simulink model "LRMate200Experimentor_RobotState"  (R2015b)
settings: Solver=FixedStepDiscrete  StartTime=0.0  StopTime=10.0  FixedStep=si.SolverTimeStep  RelTol=1e-3
model workspace (MATLAB code in the model file):
  | rsi = evalin('base', 'si.ri{1}');
undefined symbols (not defined in the file or in its folder): si
libraries: xpcethercatlib x171
(part 2 of 2)

== system LRMate200Experimentor_RobotState/Not Used/DSA System Variant/DSA System (Robot 2)/EtherCAT DSA CurrentOut ==
  FromDSA J1Current : xpcethercatlib/EtherCAT PDO Receive  Priority=2  sig_name=Box 3 (Degital Servo Adapter).HS-IN-AX01.AX01-HSI03  sig_offset=4968  sig_type=int16  type_size=16  sig_dim=1  device_id=0  sample_time=0.000250
  FromDSA J2Current : xpcethercatlib/EtherCAT PDO Receive  Priority=2  sig_name=Box 3 (Degital Servo Adapter).HS-IN-AX02.AX02-HSI03  sig_offset=5224  sig_type=int16  type_size=16  sig_dim=1  device_id=0  sample_time=0.000250
  FromDSA J3Current : xpcethercatlib/EtherCAT PDO Receive  Priority=2  sig_name=Box 3 (Degital Servo Adapter).HS-IN-AX03.AX03-HSI03  sig_offset=5480  sig_type=int16  type_size=16  sig_dim=1  device_id=0  sample_time=0.000250
  FromDSA J4Current : xpcethercatlib/EtherCAT PDO Receive  Priority=2  sig_name=Box 3 (Degital Servo Adapter).HS-IN-AX04.AX04-HSI03  sig_offset=5736  sig_type=int16  type_size=16  sig_dim=1  device_id=0  sample_time=0.000250
  FromDSA J5Current : xpcethercatlib/EtherCAT PDO Receive  Priority=2  sig_name=Box 4 (Degital Servo Adapter).HS-IN-AX01.AX01-HSI03  sig_offset=7272  sig_type=int16  type_size=16  sig_dim=1  device_id=0  sample_time=0.000250
  FromDSA J6Current : xpcethercatlib/EtherCAT PDO Receive  Priority=2  sig_name=Box 4 (Degital Servo Adapter).HS-IN-AX02.AX02-HSI03  sig_offset=7528  sig_type=int16  type_size=16  sig_dim=1  device_id=0  sample_time=0.000250
  Mux : Mux  Inputs=6
  Rate Transition : RateTransition  OutPortSampleTime=si.tsv
  CurrentOut : Outport
  wires:
  FromDSA J6Current/1 -> Mux/6
  FromDSA J4Current/1 -> Mux/4
  FromDSA J2Current/1 -> Mux/2
  FromDSA J5Current/1 -> Mux/5
  FromDSA J3Current/1 -> Mux/3
  FromDSA J1Current/1 -> Mux/1
  Mux/1 -> Rate Transition/1
  Rate Transition/1 -> CurrentOut/1

== system LRMate200Experimentor_RobotState/Not Used/DSA System Variant/DSA System (Robot 2)/EtherCAT DSA IniPos ==
  FromDSA J1IniPos : xpcethercatlib/EtherCAT PDO Receive  Priority=2  sig_name=Box 3 (Degital Servo Adapter).NS-IN-AX01.AX01-NSI02  sig_offset=6232  sig_type=int32  type_size=32  sig_dim=1  device_id=0  sample_time=0.000250
  FromDSA J2IniPos : xpcethercatlib/EtherCAT PDO Receive  Priority=2  sig_name=Box 3 (Degital Servo Adapter).NS-IN-AX02.AX02-NSI02  sig_offset=6424  sig_type=int32  type_size=32  sig_dim=1  device_id=0  sample_time=0.000250
  FromDSA J3IniPos : xpcethercatlib/EtherCAT PDO Receive  Priority=2  sig_name=Box 3 (Degital Servo Adapter).NS-IN-AX03.AX03-NSI02  sig_offset=6616  sig_type=int32  type_size=32  sig_dim=1  device_id=0  sample_time=0.000250
  FromDSA J4IniPos : xpcethercatlib/EtherCAT PDO Receive  Priority=2  sig_name=Box 3 (Degital Servo Adapter).NS-IN-AX04.AX04-NSI02  sig_offset=6808  sig_type=int32  type_size=32  sig_dim=1  device_id=0  sample_time=0.000250
  FromDSA J5IniPos : xpcethercatlib/EtherCAT PDO Receive  Priority=2  sig_name=Box 4 (Degital Servo Adapter).NS-IN-AX01.AX01-NSI02  sig_offset=8536  sig_type=int32  type_size=32  sig_dim=1  device_id=0  sample_time=0.000250
  FromDSA J6IniPos : xpcethercatlib/EtherCAT PDO Receive  Priority=2  sig_name=Box 4 (Degital Servo Adapter).NS-IN-AX02.AX02-NSI02  sig_offset=8728  sig_type=int32  type_size=32  sig_dim=1  device_id=0  sample_time=0.000250
  Mux : Mux  Inputs=6
  Rate Transition : RateTransition  OutPortSampleTime=si.tsv
  ini_pos : Outport
  wires:
  FromDSA J6IniPos/1 -> Mux/6
  FromDSA J4IniPos/1 -> Mux/4
  FromDSA J2IniPos/1 -> Mux/2
  FromDSA J5IniPos/1 -> Mux/5
  FromDSA J3IniPos/1 -> Mux/3
  FromDSA J1IniPos/1 -> Mux/1
  Mux/1 -> Rate Transition/1
  Rate Transition/1 -> ini_pos/1

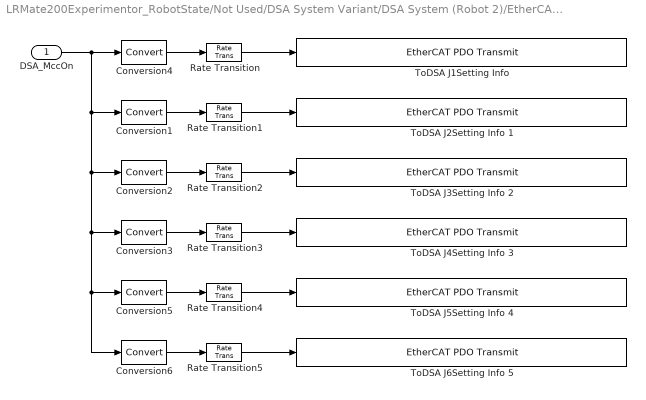
== system LRMate200Experimentor_RobotState/Not Used/DSA System Variant/DSA System (Robot 2)/EtherCAT DSA MccOn ==
  DSA_MccOn : Inport
  Conversion{1..6} (6 alike) : DataTypeConversion
  Rate Transition{,1..5} (6 alike) : RateTransition
  "ToDSA J1Setting Info " : xpcethercatlib/EtherCAT PDO Transmit   Priority=3  sig_name=Box 3 (Degital Servo Adapter).NS-OUT-AX01.AX01-NSO03  sig_offset=6248  sig_type=uint16  type_size=16  sig_dim=1  device_id=0  sample_time=0.000250
  ToDSA J2Setting Info 1 : xpcethercatlib/EtherCAT PDO Transmit   Priority=3  sig_name=Box 3 (Degital Servo Adapter).NS-OUT-AX02.AX02-NSO03  sig_offset=6504  sig_type=uint16  type_size=16  sig_dim=1  device_id=0  sample_time=0.000250
  ToDSA J3Setting Info 2 : xpcethercatlib/EtherCAT PDO Transmit   Priority=3  sig_name=Box 3 (Degital Servo Adapter).NS-OUT-AX03.AX03-NSO03  sig_offset=6760  sig_type=uint16  type_size=16  sig_dim=1  device_id=0  sample_time=0.000250
  ToDSA J4Setting Info 3 : xpcethercatlib/EtherCAT PDO Transmit   Priority=3  sig_name=Box 3 (Degital Servo Adapter).NS-OUT-AX04.AX04-NSO03  sig_offset=7016  sig_type=uint16  type_size=16  sig_dim=1  device_id=0  sample_time=0.000250
  ToDSA J5Setting Info 4 : xpcethercatlib/EtherCAT PDO Transmit   Priority=3  sig_name=Box 4 (Degital Servo Adapter).NS-OUT-AX01.AX01-NSO03  sig_offset=8552  sig_type=uint16  type_size=16  sig_dim=1  device_id=0  sample_time=0.000250
  ToDSA J6Setting Info 5 : xpcethercatlib/EtherCAT PDO Transmit   Priority=3  sig_name=Box 4 (Degital Servo Adapter).NS-OUT-AX02.AX02-NSO03  sig_offset=8808  sig_type=uint16  type_size=16  sig_dim=1  device_id=0  sample_time=0.000250
  wires:
  Rate Transition/1 -> "ToDSA J1Setting Info "/1
  Conversion4/1 -> Rate Transition/1
  DSA_MccOn/1 -> Conversion6/1, Conversion5/1, Conversion3/1, Conversion2/1, Conversion1/1, Conversion4/1
  Rate Transition1/1 -> ToDSA J2Setting Info 1/1
  Conversion1/1 -> Rate Transition1/1
  Rate Transition2/1 -> ToDSA J3Setting Info 2/1
  Conversion2/1 -> Rate Transition2/1
  Rate Transition3/1 -> ToDSA J4Setting Info 3/1
  Conversion3/1 -> Rate Transition3/1
  Rate Transition4/1 -> ToDSA J5Setting Info 4/1
  Conversion5/1 -> Rate Transition4/1
  Rate Transition5/1 -> ToDSA J6Setting Info 5/1
  Conversion6/1 -> Rate Transition5/1

== system LRMate200Experimentor_RobotState/Not Used/DSA System Variant/DSA System (Robot 2)/EtherCAT DSA PosOut ==
  FromDSA J1Pos : xpcethercatlib/EtherCAT PDO Receive  Priority=2  sig_name=Box 3 (Degital Servo Adapter).HS-IN-AX01.AX01-HSI12  sig_offset=5112  sig_type=int32  type_size=32  sig_dim=1  device_id=0  sample_time=0.000250
  FromDSA J2Pos : xpcethercatlib/EtherCAT PDO Receive  Priority=2  sig_name=Box 3 (Degital Servo Adapter).HS-IN-AX02.AX02-HSI12  sig_offset=5368  sig_type=int32  type_size=32  sig_dim=1  device_id=0  sample_time=0.000250
  FromDSA J3Pos : xpcethercatlib/EtherCAT PDO Receive  Priority=2  sig_name=Box 3 (Degital Servo Adapter).HS-IN-AX03.AX03-HSI12  sig_offset=5624  sig_type=int32  type_size=32  sig_dim=1  device_id=0  sample_time=0.000250
  FromDSA J4Pos : xpcethercatlib/EtherCAT PDO Receive  Priority=2  sig_name=Box 3 (Degital Servo Adapter).HS-IN-AX04.AX04-HSI12  sig_offset=5880  sig_type=int32  type_size=32  sig_dim=1  device_id=0  sample_time=0.000250
  FromDSA J5Pos : xpcethercatlib/EtherCAT PDO Receive  Priority=2  sig_name=Box 4 (Degital Servo Adapter).HS-IN-AX01.AX01-HSI12  sig_offset=7416  sig_type=int32  type_size=32  sig_dim=1  device_id=0  sample_time=0.000250
  FromDSA J6Pos : xpcethercatlib/EtherCAT PDO Receive  Priority=2  sig_name=Box 4 (Degital Servo Adapter).HS-IN-AX02.AX02-HSI12  sig_offset=7672  sig_type=int32  type_size=32  sig_dim=1  device_id=0  sample_time=0.000250
  Mux : Mux  Inputs=6
  Rate Transition : RateTransition  OutPortSampleTime=si.tsv
  PosOut : Outport
  wires:
  FromDSA J6Pos/1 -> Mux/6
  FromDSA J4Pos/1 -> Mux/4
  FromDSA J2Pos/1 -> Mux/2
  FromDSA J5Pos/1 -> Mux/5
  FromDSA J3Pos/1 -> Mux/3
  FromDSA J1Pos/1 -> Mux/1
  Mux/1 -> Rate Transition/1
  Rate Transition/1 -> PosOut/1

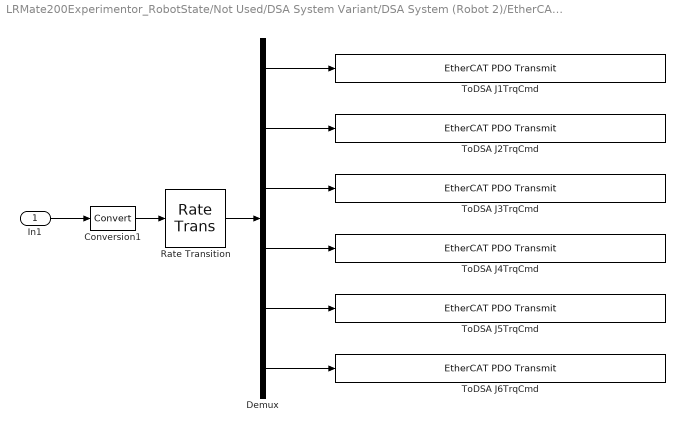
== system LRMate200Experimentor_RobotState/Not Used/DSA System Variant/DSA System (Robot 2)/EtherCAT DSA TrqCmd ==
  In1 : Inport
  Conversion1 : DataTypeConversion
  Demux : Demux  Outputs=6
  Rate Transition : RateTransition
  "ToDSA J1TrqCmd " : xpcethercatlib/EtherCAT PDO Transmit   Priority=3  sig_name=Box 3 (Degital Servo Adapter).HS-OUT-AX01.AX01-HSO04  sig_offset=4984  sig_type=int16  type_size=16  sig_dim=1  device_id=0  sample_time=0.000250
  ToDSA J2TrqCmd : xpcethercatlib/EtherCAT PDO Transmit   Priority=3  sig_name=Box 3 (Degital Servo Adapter).HS-OUT-AX02.AX02-HSO04  sig_offset=5240  sig_type=int16  type_size=16  sig_dim=1  device_id=0  sample_time=0.000250
  ToDSA J3TrqCmd : xpcethercatlib/EtherCAT PDO Transmit   Priority=3  sig_name=Box 3 (Degital Servo Adapter).HS-OUT-AX03.AX03-HSO04  sig_offset=5496  sig_type=int16  type_size=16  sig_dim=1  device_id=0  sample_time=0.000250
  ToDSA J4TrqCmd : xpcethercatlib/EtherCAT PDO Transmit   Priority=3  sig_name=Box 3 (Degital Servo Adapter).HS-OUT-AX04.AX04-HSO04  sig_offset=5752  sig_type=int16  type_size=16  sig_dim=1  device_id=0  sample_time=0.000250
  ToDSA J5TrqCmd : xpcethercatlib/EtherCAT PDO Transmit   Priority=3  sig_name=Box 4 (Degital Servo Adapter).HS-OUT-AX01.AX01-HSO04  sig_offset=7288  sig_type=int16  type_size=16  sig_dim=1  device_id=0  sample_time=0.000250
  ToDSA J6TrqCmd : xpcethercatlib/EtherCAT PDO Transmit   Priority=3  sig_name=Box 4 (Degital Servo Adapter).HS-OUT-AX02.AX02-HSO04  sig_offset=7544  sig_type=int16  type_size=16  sig_dim=1  device_id=0  sample_time=0.000250
  wires:
  In1/1 -> Conversion1/1
  Conversion1/1 -> Rate Transition/1
  Rate Transition/1 -> Demux/1
  Demux/1 -> "ToDSA J1TrqCmd "/1
  Demux/2 -> ToDSA J2TrqCmd/1
  Demux/3 -> ToDSA J3TrqCmd/1
  Demux/4 -> ToDSA J4TrqCmd/1
  Demux/5 -> ToDSA J5TrqCmd/1
  Demux/6 -> ToDSA J6TrqCmd/1

== system LRMate200Experimentor_RobotState/Not Used/DSA System Variant/DSA System (Robot 2)/EtherCAT DSA TrqCmdOut ==
  FromDSA J1TrqCmd : xpcethercatlib/EtherCAT PDO Receive  Priority=2  sig_name=Box 3 (Degital Servo Adapter).HS-IN-AX01.AX01-HSI02  sig_offset=4952  sig_type=int16  type_size=16  sig_dim=1  device_id=0  sample_time=0.000250
  FromDSA J2TrqCmd : xpcethercatlib/EtherCAT PDO Receive  Priority=2  sig_name=Box 3 (Degital Servo Adapter).HS-IN-AX02.AX02-HSI02  sig_offset=5208  sig_type=int16  type_size=16  sig_dim=1  device_id=0  sample_time=0.000250
  FromDSA J3TrqCmd2 : xpcethercatlib/EtherCAT PDO Receive  Priority=2  sig_name=Box 3 (Degital Servo Adapter).HS-IN-AX03.AX03-HSI02  sig_offset=5464  sig_type=int16  type_size=16  sig_dim=1  device_id=0  sample_time=0.000250
  FromDSA J4TrqCmd3 : xpcethercatlib/EtherCAT PDO Receive  Priority=2  sig_name=Box 3 (Degital Servo Adapter).HS-IN-AX04.AX04-HSI02  sig_offset=5720  sig_type=int16  type_size=16  sig_dim=1  device_id=0  sample_time=0.000250
  FromDSA J5TrqCmd4 : xpcethercatlib/EtherCAT PDO Receive  Priority=2  sig_name=Box 4 (Degital Servo Adapter).HS-IN-AX01.AX01-HSI02  sig_offset=7256  sig_type=int16  type_size=16  sig_dim=1  device_id=0  sample_time=0.000250
  FromDSA J6TrqCmd5 : xpcethercatlib/EtherCAT PDO Receive  Priority=2  sig_name=Box 4 (Degital Servo Adapter).HS-IN-AX02.AX02-HSI02  sig_offset=7512  sig_type=int16  type_size=16  sig_dim=1  device_id=0  sample_time=0.000250
  Mux : Mux  Inputs=6
  Rate Transition : RateTransition  OutPortSampleTime=si.tsv
  TrqCmdOut : Outport
  wires:
  FromDSA J6TrqCmd5/1 -> Mux/6
  FromDSA J4TrqCmd3/1 -> Mux/4
  FromDSA J2TrqCmd/1 -> Mux/2
  FromDSA J5TrqCmd4/1 -> Mux/5
  FromDSA J3TrqCmd2/1 -> Mux/3
  FromDSA J1TrqCmd/1 -> Mux/1
  Mux/1 -> Rate Transition/1
  Rate Transition/1 -> TrqCmdOut/1

== system LRMate200Experimentor_RobotState/Not Used/DSA System Variant/DSA System (Robot 2)/EtherCAT DSA TrqLimit ==
  In1 : Inport
  Conversion1 : DataTypeConversion
  Demux : Demux  Outputs=6
  "ToDSA J1TrqLimit " : xpcethercatlib/EtherCAT PDO Transmit   Priority=3  sig_name=Box 3 (Degital Servo Adapter).HS-OUT-AX01.AX01-HSO05  sig_offset=5000  sig_type=int16  type_size=16  sig_dim=1  device_id=0  sample_time=0.000250
  ToDSA J2TrqLimit : xpcethercatlib/EtherCAT PDO Transmit   Priority=3  sig_name=Box 3 (Degital Servo Adapter).HS-OUT-AX02.AX02-HSO05  sig_offset=5256  sig_type=int16  type_size=16  sig_dim=1  device_id=0  sample_time=0.000250
  ToDSA J3TrqLimit : xpcethercatlib/EtherCAT PDO Transmit   Priority=3  sig_name=Box 3 (Degital Servo Adapter).HS-OUT-AX03.AX03-HSO05  sig_offset=5512  sig_type=int16  type_size=16  sig_dim=1  device_id=0  sample_time=0.000250
  ToDSA J4TrqLimit : xpcethercatlib/EtherCAT PDO Transmit   Priority=3  sig_name=Box 3 (Degital Servo Adapter).HS-OUT-AX04.AX04-HSO05  sig_offset=5768  sig_type=int16  type_size=16  sig_dim=1  device_id=0  sample_time=0.000250
  ToDSA J5TrqLimit : xpcethercatlib/EtherCAT PDO Transmit   Priority=3  sig_name=Box 4 (Degital Servo Adapter).HS-OUT-AX01.AX01-HSO05  sig_offset=7304  sig_type=int16  type_size=16  sig_dim=1  device_id=0  sample_time=0.000250
  ToDSA J6TrqLimit : xpcethercatlib/EtherCAT PDO Transmit   Priority=3  sig_name=Box 4 (Degital Servo Adapter).HS-OUT-AX02.AX02-HSO05  sig_offset=7560  sig_type=int16  type_size=16  sig_dim=1  device_id=0  sample_time=0.000250
  wires:
  In1/1 -> Conversion1/1
  Conversion1/1 -> Demux/1
  Demux/1 -> "ToDSA J1TrqLimit "/1
  Demux/2 -> ToDSA J2TrqLimit/1
  Demux/3 -> ToDSA J3TrqLimit/1
  Demux/4 -> ToDSA J4TrqLimit/1
  Demux/5 -> ToDSA J5TrqLimit/1
  Demux/6 -> ToDSA J6TrqLimit/1

== system LRMate200Experimentor_RobotState/Not Used/DSA System Variant/DSA System (Robot 2)/EtherCAT DSA VelOut ==
  FromDSA J1Vel : xpcethercatlib/EtherCAT PDO Receive  Priority=2  sig_name=Box 3 (Degital Servo Adapter).HS-IN-AX01.AX01-HSI10  sig_offset=5080  sig_type=int32  type_size=32  sig_dim=1  device_id=0  sample_time=0.000250
  FromDSA J2Vel : xpcethercatlib/EtherCAT PDO Receive  Priority=2  sig_name=Box 3 (Degital Servo Adapter).HS-IN-AX02.AX02-HSI10  sig_offset=5336  sig_type=int32  type_size=32  sig_dim=1  device_id=0  sample_time=0.000250
  FromDSA J3Vel : xpcethercatlib/EtherCAT PDO Receive  Priority=2  sig_name=Box 3 (Degital Servo Adapter).HS-IN-AX03.AX03-HSI10  sig_offset=5592  sig_type=int32  type_size=32  sig_dim=1  device_id=0  sample_time=0.000250
  FromDSA J4Vel : xpcethercatlib/EtherCAT PDO Receive  Priority=2  sig_name=Box 3 (Degital Servo Adapter).HS-IN-AX04.AX04-HSI10  sig_offset=5848  sig_type=int32  type_size=32  sig_dim=1  device_id=0  sample_time=0.000250
  FromDSA J5Vel : xpcethercatlib/EtherCAT PDO Receive  Priority=2  sig_name=Box 4 (Degital Servo Adapter).HS-IN-AX01.AX01-HSI10  sig_offset=7384  sig_type=int32  type_size=32  sig_dim=1  device_id=0  sample_time=0.000250
  FromDSA J6Vel : xpcethercatlib/EtherCAT PDO Receive  Priority=2  sig_name=Box 4 (Degital Servo Adapter).HS-IN-AX02.AX02-HSI10  sig_offset=7640  sig_type=int32  type_size=32  sig_dim=1  device_id=0  sample_time=0.000250
  Mux : Mux  Inputs=6
  Rate Transition : RateTransition  OutPortSampleTime=si.tsv
  VelOut : Outport
  wires:
  FromDSA J6Vel/1 -> Mux/6
  FromDSA J4Vel/1 -> Mux/4
  FromDSA J2Vel/1 -> Mux/2
  FromDSA J5Vel/1 -> Mux/5
  FromDSA J3Vel/1 -> Mux/3
  FromDSA J1Vel/1 -> Mux/1
  Rate Transition/1 -> VelOut/1
  Mux/1 -> Rate Transition/1

== matlab function LRMate200Experimentor_RobotState/MATLAB Function ==
  data: DH input; T_B2W input; T output; JointPos input; J_M output; J_T output; TCP_Pos output; TCP_Pos_W output; Tilt_Angle output
function [T, J_M, J_T, TCP_Pos, TCP_Pos_W, Tilt_Angle] = fkine_robot2workpice(DH, T_B2W, JointPos)

% input:  DH parameter for robots, tool, and workpiece, current Joint Position (rad)
% output: Transformation Matrix and Jabobian Matrix

% Changed J_M to World Frame, DH to include tool and workpiece parameters  
% Order: J1, J2, ..., Jn, Tool, Workpiece
% -- Wenjie Chen, 2016/06/23

axis_num = size(DH,2)-2;    % The last two columns are for tool and workpiece

%% Transformation Matrix for each joint and tool and workpiece
JointPos = [JointPos; 0; 0];  % Add 0 as aritifical joint pos for tool and workpiece
Tr = eye(4,4);
T = nan(4,4,size(DH,2));
for i=1:size(DH,2)
    q = JointPos(i) + DH(1,i);
    Tr = Tr * [cos(q)      -sin(q)*cos(DH(4,i))    sin(q)*sin(DH(4,i))      DH(3,i)*cos(q);
               sin(q)      cos(q)*cos(DH(4,i))     -cos(q)*sin(DH(4,i))     sin(q)*DH(3,i);
               0           sin(DH(4,i))            cos(DH(4,i))             DH(2,i);
               0           0                       0                        1];
    T(:,:,i) = Tr;
end

%% Jacobian Matrix of the TCP      
J = nan(6,axis_num);

J(:,1) = [cross( [0;0;0] - T(1:3,4,axis_num+1), [0;0;1] ); [0;0;1]];
for i=1:axis_num-1
    J(:,i+1)=[cross( T(1:3,4,i) - T(1:3,4,axis_num+1), T(1:3,3,i) ); T(1:3,3,i)];
end

%% JacobianM Matrix at world frame
% Changed J_M to World Frame  -- Wenjie Chen, 2016/06/23
R_B2W = T_B2W(1:3,1:3);
J_M = blkdiag(R_B2W, R_B2W)*J;

%% JacobianT Matrix at tool frame
R_T2B = T(1:3,1:3,axis_num+1);
J_T = blkdiag(R_T2B', R_T2B')*J;

%% TCP position 
TCP_Pos = T(1:3,4,axis_num+1);
TCP_Pos_W0 = T_B2W * T(1:4,4,axis_num+1);
TCP_Pos_W = TCP_Pos_W0(1:3);

%% Tool Tilted Angle
Tilt_Angle = acosd(T(1:3,3,axis_num+1)'*[0;0;-1]);

end

== matlab function LRMate200Experimentor_RobotState/Not Used/MATLAB Function ==
  data: DH input; ToolDH input; Bar_DH input; T_B2W input; T output; JointPos input; J_M output; J_T output; TCP_Pos output; Tilt_Angle output
function [T, J_M, J_T,TCP_Pos,Tilt_Angle] = fkine_msc_bar(DH, ToolDH, Bar_DH, T_B2W, JointPos)

% input:  DH parameter for robots, Tool DH Parameter, current Joint Position (rad)
% output: Transformation Matrix and Jabobian Matrix

% Changed J_M to World Frame  -- Wenjie Chen, 2016/06/23

%% Transformation Matrix for the first 6 joint frame
Tr = eye(4,4);
T = nan(4,4,8);
for i=1:6
    q = JointPos(i) + DH(1,i);
    Tr = Tr * [cos(q)      -sin(q)*cos(DH(4,i))    sin(q)*sin(DH(4,i))      DH(3,i)*cos(q);
               sin(q)      cos(q)*cos(DH(4,i))     -cos(q)*sin(DH(4,i))     sin(q)*DH(3,i);
               0           sin(DH(4,i))            cos(DH(4,i))             DH(2,i);
               0           0                       0                        1];
    T(:,:,i) = Tr;
end

%% Transformation Matrix for the Tool Frame
q = 0 + ToolDH(1);
T(:,:,7) = T(:,:,6) * [cos(q)     -sin(q)*cos(ToolDH(4))    sin(q)*sin(ToolDH(4))    ToolDH(3)*cos(q);
                       sin(q)     cos(q)*cos(ToolDH(4))     -cos(q)*sin(ToolDH(4))   sin(q)*ToolDH(3);
                       0          sin(ToolDH(4))            cos(ToolDH(4))           ToolDH(2);
                       0          0                         0                        1];
%% Transformation matrix for handling bar
q = 0 + Bar_DH(1);
T(:,:,8) = T(:,:,6) * [cos(q)     -sin(q)*cos(Bar_DH(4))    sin(q)*sin(Bar_DH(4))    Bar_DH(3)*cos(q);
                       sin(q)     cos(q)*cos(Bar_DH(4))     -cos(q)*sin(Bar_DH(4))   sin(q)*Bar_DH(3);
                       0          sin(Bar_DH(4))            cos(Bar_DH(4))           Bar_DH(2);
                       0          0                         0                        1];
%% Jacobian Matrix      
J = nan(6,6);

J(:,1) = [cross( [0;0;0] - T(1:3,4,7), [0;0;1] ); [0;0;1]];
for i=1:5
    J(:,i+1)=[cross( T(1:3,4,i) - T(1:3,4,7), T(1:3,3,i) ); T(1:3,3,i)];
end

%% JacobianM Matrix
% Changed J_M to World Frame  -- Wenjie Chen, 2016/06/23
R_B2W = T_B2W(1:3,1:3);
J_M = blkdiag(R_B2W, R_B2W)*J;

%% JacobianT Matrix
R_T2B = T(1:3,1:3,7);
J_T = blkdiag(R_T2B', R_T2B')*J;

%% TCP position 
TCP_Pos = T(1:3,4,7);

%% Tool Tilted Angle
Tilt_Angle = acosd(T(1:3,3,7)'*[0;0;-1]);

end

== matlab function LRMate200Experimentor_RobotState/Not Used/MATLAB Function1 ==
  data: DH input; ToolDH input; T output; JointPos input; J output; J_T output; TCP_Pos output; Tilt_Angle output
function [T,J, J_T,TCP_Pos,Tilt_Angle] = fkine_msc(DH, ToolDH, JointPos)

% input:  DH parameter for robots, Tool DH Parameter, current Joint Position (rad)
% output: Transformation Matrix and Jabobian Matrix

%% Transformation Matrix for the first 6 joint frame
Tr = eye(4,4);
T = nan(4,4,7);
for i=1:6
    q = JointPos(i) + DH(1,i);
    Tr = Tr * [cos(q)      -sin(q)*cos(DH(4,i))    sin(q)*sin(DH(4,i))      DH(3,i)*cos(q);
               sin(q)      cos(q)*cos(DH(4,i))     -cos(q)*sin(DH(4,i))     sin(q)*DH(3,i);
               0           sin(DH(4,i))            cos(DH(4,i))             DH(2,i);
               0           0                       0                        1];
    T(:,:,i) = Tr;
end

%% Transformation Matrix for the Tool Frame
q = 0 + ToolDH(1);
T(:,:,7) = T(:,:,6) * [cos(q)     -sin(q)*cos(ToolDH(4))    sin(q)*sin(ToolDH(4))    ToolDH(3)*cos(q);
                       sin(q)     cos(q)*cos(ToolDH(4))     -cos(q)*sin(ToolDH(4))   sin(q)*ToolDH(3);
                       0          sin(ToolDH(4))            cos(ToolDH(4))           ToolDH(2);
                       0          0                         0                        1];
                   
%% Jacobian Matrix      
J = nan(6,6);

J(:,1) = [cross( [0;0;0] - T(1:3,4,7), [0;0;1] ); [0;0;1]];
for i=1:5
    J(:,i+1)=[cross( T(1:3,4,i) - T(1:3,4,7), T(1:3,3,i) ); T(1:3,3,i)];
end

%% JacobianT Matrix
R_T2B = T(1:3,1:3,7);
J_T = blkdiag(R_T2B', R_T2B')*J;

%% TCP position 
TCP_Pos = T(1:3,4,7);

%% Tool Tilted Angle
Tilt_Angle = acosd(T(1:3,3,7)'*[0;0;-1]);


end
